simulink library "inp"  (Simulink 7.4)
settings: Solver=ode45  StartTime=0.0  StopTime=10.0  RelTol=1e-3
undefined symbols (not defined in the file): AINP_BrkPedalInterp_X_bar, C_TASK_10MS_S, ENUM_SHIFTER_D, ENUM_SHIFTER_N, ENUM_SHIFTER_P, ENUM_SHIFTER_R, KINP_BonnetCloseVehSpdThre_kph, KINP_EDUCoolantTempFilTm_s, KINP_EDUOilPressureFilTm_s, KINP_EDUOilTempFilTm_s, KINP_EDUSynchDisp_mm, KINP_EDUSynchPosnPWMDC_pct_LowerLimit, KINP_EDUSynchPosnPWMDC_pct_ovrdflg, KINP_EDUSynchPosnPWMDC_pct_ovrdval, KINP_EDUSynchPosnPWMDC_pct_UpperLimit, KINP_ShifterPosConfirmD_s, KINP_ShifterPosConfirmN_s, KINP_ShifterPosConfirmP_s, KINP_ShifterPosConfirmR_s, KINP_SingleAccPedalFltRateLim_pct, KINP_TMSpd2VehSpdSigNeg_rpm, KINP_TMSpd2VehSpdSigPos_rpm, KINP_ValidCheck_EDUSynchPosnPWMDC_dec, KINP_ValidCheck_EDUSynchPosnPWMDC_inc, KINP_ValidCheck_EDUSynchPosnPWMDC_lim, KINP_VehSpdSigKeepThres_kph, KPH2MPS, MIN2SEC, MINP_BrkPedalInterp_pct, MPS2KPH, PI, seat_version_control_block_callbacks, TIRE_RADIUS
libraries: inp_lib x166, hcu_lib x4, simulink x1
(part 9 of 9)

== system inp/INP/INP_10MS/Message (10ms) SCU_HSC_FrP00/Subsystem ==
  VINP_ShifterPosRaw_enum : Inport  OutDataType=fixdt(1, 16)  OutScaling=2^0
  Constant10 : Constant  Value=ENUM_SHIFTER_N  OutDataType=fixdt(1, 16)  OutScaling=2^0
  Constant11 : Constant  Value=ENUM_SHIFTER_R  OutDataType=fixdt(1, 16)  OutScaling=2^0
  Constant22 : Constant  Value=ENUM_SHIFTER_D  OutDataType=fixdt(1, 16)  OutScaling=2^0
  Constant23 : Constant  Value=ENUM_SHIFTER_P  OutDataType=fixdt(1, 16)  OutScaling=2^0
  Constant24 : Constant  Value=KINP_ShifterPosConfirmN_s  OutDataType=fixdt(1, 16)  OutScaling=2^0
  Constant25 : Constant  Value=KINP_ShifterPosConfirmR_s  OutDataType=fixdt(1, 16)  OutScaling=2^0
  Constant26 : Constant  Value=KINP_ShifterPosConfirmD_s  OutDataType=fixdt(1, 16)  OutScaling=2^0
  Constant27 : Constant  Value=KINP_ShifterPosConfirmP_s  OutDataType=fixdt(1, 16)  OutScaling=2^0
  Constant28 : Constant  Value=C_TASK_10MS_S  OutDataTypeMode=single  OutDataType=fixdt(1, 16)  OutScaling=2^0  OutDataTypeStr=single
  Relational Operator{5,10..12} (4 alike) : RelationalOperator  Operator===  LogicOutDataTypeMode=boolean  LogicDataType=fixdt(0, 8)  OutDataTypeStr=boolean
  Relational Operator4 : RelationalOperator  Operator=~=  LogicOutDataTypeMode=boolean  LogicDataType=fixdt(0, 8)  OutDataTypeStr=boolean
  Switch{4,9..12} (5 alike) : Switch  Criteria=u2 ~= 0  Threshold=0.5  OutDataType=fixdt(1, 16)  OutScaling=2^0
  Terminator : Terminator
  Timer : Subsystem
  Unit Delay5 : UnitDelay  X0=ENUM_SHIFTER_P  SampleTime=-1
      settings: AttributesFormatString=Initial value=ENUM_SHIFTER_P
  Unit Delay6 : UnitDelay  SampleTime=-1
  Unit Delay7 : UnitDelay  X0=ENUM_SHIFTER_P  SampleTime=-1
      settings: AttributesFormatString=Initial value=ENUM_SHIFTER_P
  VINP_ShifterPos_enum : Outport  OutDataType=fixdt(1, 16)  OutScaling=2^0
  wires:
  VINP_ShifterPosRaw_enum/1 -> Relational Operator12/1, Relational Operator5/1, Relational Operator11/1, Unit Delay5/1, Relational Operator4/1, Relational Operator10/1, Switch12/1
  Unit Delay5/1 -> Relational Operator4/2
  Constant10/1 -> Relational Operator5/2
  Constant11/1 -> Relational Operator10/2
  Constant22/1 -> Relational Operator11/2
  Constant23/1 -> Relational Operator12/2
  Constant24/1 -> Switch11/1
  Relational Operator5/1 -> Switch11/2
  Constant25/1 -> Switch10/1
  Relational Operator10/1 -> Switch10/2
  Constant26/1 -> Switch4/1
  Relational Operator11/1 -> Switch4/2
  Constant27/1 -> Switch9/1
  Relational Operator12/1 -> Switch9/2
  Switch10/1 -> Switch4/3
  Switch4/1 -> Switch11/3
  Switch11/1 -> Switch9/3
  Switch9/1 -> Unit Delay6/1, Timer/1(To)
  Unit Delay6/1 -> Switch10/3
  Relational Operator4/1 -> Timer/3(reset)
  Constant28/1 -> Timer/2(Ts)
  Timer/1(time) -> Terminator/1
  Timer/2(timeout) -> Switch12/2
  Switch12/1 -> Unit Delay7/1, VINP_ShifterPos_enum/1
  Unit Delay7/1 -> Switch12/3

== system inp/INP/INP_20MS/HW_HCU_20ms/filter ==
  VINP_EDUOilPressureRaw_bar : Inport  OutDataType=sfix(16)  OutScaling=2^0
  Constant : Constant  Value=0.02  OutDataTypeMode=single  OutDataType=fixdt(1, 16)  OutScaling=2^0  OutDataTypeStr=single
  Constant1 : Constant  Value=KINP_EDUOilPressureFilTm_s  OutDataTypeMode=single  OutDataType=fixdt(1, 16)  OutScaling=2^0  OutDataTypeStr=single
  First_Order_Filter : hcu_lib/First_Order_Filter  SystemSampleTime=-1
  VINP_EDUOilPressure_bar : Outport  OutDataType=sfix(16)  OutScaling=2^0
  wires:
  Constant1/1 -> First_Order_Filter/2
  Constant/1 -> First_Order_Filter/3
  First_Order_Filter/1 -> VINP_EDUOilPressure_bar/1
  VINP_EDUOilPressureRaw_bar/1 -> First_Order_Filter/1

== system inp/INP/INP_5MS/HW_HCU_5ms/Subsys VINP_EDUSynchPosnPWMDC_pct ==
  note: Function:
      | 1. Calibration override
      | 2. Valid signal debounce and default value selection
      | 3. High/Low saturation
      | Applicable for:
      | 1. Hardwire analog signals (with corresponding valid flag)
  SigIn : Inport  OutDataType=fixdt(1, 16)  OutScaling=2^0
  SigValidRaw : Inport  Port=2  OutDataType=fixdt(1, 16)  OutScaling=2^0
  srv_ovrdflg : Inport  Port=3  OutDataType=fixdt(1, 16)  OutScaling=2^0
  srv_ovrdval : Inport  Port=4  OutDataType=fixdt(1, 16)  OutScaling=2^0
  Data Type Conversion : DataTypeConversion  OutDataType=fixdt(1, 16)  OutScaling=2^0
  Data Type Conversion1 : DataTypeConversion  OutDataType=fixdt(1, 16)  OutScaling=2^0
  Logical Operator : Logic  Operator=NOT  Inputs=1  AllPortsSameDT=off  OutDataTypeMode=boolean  LogicDataType=fixdt(0, 8)  OutDataTypeStr=boolean
  Logical Operator1 : Logic  Operator=NOT  Inputs=1  AllPortsSameDT=off  OutDataTypeMode=boolean  LogicDataType=fixdt(0, 8)  OutDataTypeStr=boolean
  Logical Operator2 : Logic  Operator=OR  AllPortsSameDT=off  OutDataTypeMode=boolean  OutDataTypeStr=boolean
  MinMax : MinMax  Inputs=2  OutDataType=fixdt(1, 16)  OutScaling=2^0
  MinMax1 : MinMax  Function=max  Inputs=2  OutDataType=fixdt(1, 16)  OutScaling=2^0
  Switch1 : Switch  Criteria=u2 ~= 0  OutDataType=fixdt(1, 16)  OutScaling=2^0
  Switch2 : Switch  Criteria=u2 ~= 0  OutDataType=fixdt(1, 16)  OutScaling=2^0
  Switch3 : Switch  Criteria=u2 ~= 0  Threshold=0.5  OutDataType=sfix(16)  OutScaling=2^0
  Switch4 : Switch  Criteria=u2 ~= 0  Threshold=0.5  OutDataType=sfix(16)  OutScaling=2^0
  Switch5 : Switch  Criteria=u2 ~= 0  Threshold=0.5  OutDataType=sfix(16)  OutScaling=2^0
  Terminator : Terminator
  True : Constant  OutDataTypeMode=boolean  OutDataType=sfix(16)  OutScaling=2^0  OutDataTypeStr=boolean
  Unit Delay : UnitDelay  SampleTime=-1
      settings: AttributesFormatString=Init: %<X0>
  Unit Delay1 : UnitDelay  SampleTime=-1
  rff_ctl : Stateflow chart
  sat : Constant  Value=lim  OutDataTypeMode=uint8  OutDataType=sfix(16)  OutScaling=2^0  OutDataTypeStr=uint8
  sat1 : Constant  Value=inc  OutDataTypeMode=uint8  OutDataType=sfix(16)  OutScaling=2^0  OutDataTypeStr=uint8
  sat2 : Constant  Value=dec  OutDataTypeMode=uint8  OutDataType=sfix(16)  OutScaling=2^0  OutDataTypeStr=uint8
  sat3 : Constant  Value=cal_ovrdflg  OutDataTypeMode=boolean  OutDataType=sfix(16)  OutScaling=2^0  OutDataTypeStr=boolean
  sat4 : Constant  Value=cal_ovrdval  OutDataType=sfix(16)  OutScaling=2^0  OutDataTypeStr=Inherit: Inherit via back propagation
  sat6 : Constant  Value=hi  OutDataType=sfix(16)  OutScaling=2^0  OutDataTypeStr=Inherit: Inherit via back propagation
  sat7 : Constant  Value=lo  OutDataType=sfix(16)  OutScaling=2^0  OutDataTypeStr=Inherit: Inherit via back propagation
  SigOut : Outport  OutDataType=fixdt(1, 16)  OutScaling=2^0
  SigValid : Outport  Port=2  OutDataType=fixdt(1, 16)  OutScaling=2^0
  wires:
  MinMax1/1 -> Switch4/3
  Switch2/1 -> MinMax/1
  sat6/1 -> MinMax/2
  sat7/1 -> MinMax1/2
  MinMax/1 -> MinMax1/1
  [sig_valid] -> Switch5/3
  Logical Operator/1 -> [sig_valid], Switch2/2
  Switch5/1 -> SigValid/1
  True/1 -> Switch5/1
  Logical Operator2/1 -> Switch5/2
  Switch4/1 -> Switch3/3
  Data Type Conversion/1 -> Switch4/1  "cal_ovrdval"
  srv_ovrdval/1 -> Switch3/1  "srv_ovrdval"
  sat3/1 -> Switch4/2, [cal_ovrdflg]  "cal_ovrdflg"
  srv_ovrdflg/1 -> Switch3/2, [service_ovrdflg]  "srv_ovrdflg"
  Switch3/1 -> SigOut/1, Unit Delay1/1
  [service_ovrdflg] -> Logical Operator2/1
  [cal_ovrdflg] -> Logical Operator2/2
  SigValidRaw/1 -> Logical Operator1/1, Switch1/2
  Logical Operator1/1 -> rff_ctl/4(i_fault)
  Unit Delay/1 -> Switch1/3
  Switch1/1 -> Switch2/1, Unit Delay/1
  Data Type Conversion1/1 -> Switch2/3
  rff_ctl/2(ff_count) -> Terminator/1
  rff_ctl/1(fault_flg) -> Logical Operator/1
  sat2/1 -> rff_ctl/3(dec)
  sat1/1 -> rff_ctl/2(inc)
  sat/1 -> rff_ctl/1(sat)
  SigIn/1 -> Switch1/1
  sat4/1 -> Data Type Conversion/1
  Unit Delay1/1 -> Data Type Conversion1/1

== system inp/INP/Pre-Process/BINP_ouputs_100ms/Outputs_100ms ==
  VINP_BonnetOpen_flg : Inport  OutDataType=fixdt(1, 16)  OutScaling=2^0
  BINP_rawoutputs_100ms : Inport  Port=2  OutDataType=fixdt(1, 16)  OutScaling=2^0
  Bus Creator1 : BusCreator  Inputs=5
  Bus Creator2 : BusCreator  Inputs=9
  Bus Selector1 : BusSelector  OutputSignals=BINP_ISC_HSC2_FrP05,BINP_TC_HSC2_FrP03,BINP_ISC_HSC2_FrP01,BINP_ISC_HSC2_FrP02,BINP_PMU_HSC_FrP00,BINP_SMU_HSC_FrP07,BINP_SMU_HSC_FrP00,BINP_HW_HCU_100ms
  Bus Selector2 : BusSelector  OutputSignals=BINP_SMU_HSC_FrP06.VINP_DriverDoorOpen_flg,BINP_SMU_HSC_FrP06.VINP_ATCEngOnReq_enum,BINP_SMU_HSC_FrP06.VINP_ACCompressorPower_kW,BINP_SMU_HSC_FrP06.VINP_SMUHSCFrP06Active_flg
  Bus Selector7 : BusSelector  OutputSignals=BINP_ISC_HSC2_FrP05,BINP_TC_HSC2_FrP03,BINP_ISC_HSC2_FrP01,BINP_ISC_HSC2_FrP02,BINP_PMU_HSC_FrP00,BINP_SMU_HSC_FrP07,BINP_SMU_HSC_FrP00,BINP_HW_HCU_100ms,BINP_SMU_HSC_FrP06  OutputAsBus=on
  BINP_outputs_100ms : Outport  OutDataType=fixdt(1, 16)  OutScaling=2^0
  wires:
  Bus Creator1/1 -> Bus Creator2/9  "BINP_SMU_HSC_FrP06"
  Bus Selector1/8 -> Bus Creator2/8  "<BINP_HW_HCU_100ms>"
  Bus Selector1/7 -> Bus Creator2/7  "<BINP_SMU_HSC_FrP00>"
  Bus Selector1/6 -> Bus Creator2/6  "<BINP_SMU_HSC_FrP07>"
  Bus Selector1/5 -> Bus Creator2/5  "<BINP_PMU_HSC_FrP00>"
  Bus Selector1/4 -> Bus Creator2/4  "<BINP_ISC_HSC2_FrP02>"
  Bus Selector1/3 -> Bus Creator2/3  "<BINP_ISC_HSC2_FrP01>"
  Bus Selector1/2 -> Bus Creator2/2  "<BINP_TC_HSC2_FrP03>"
  Bus Selector1/1 -> Bus Creator2/1  "<BINP_ISC_HSC2_FrP05>"
  VINP_BonnetOpen_flg/1 -> Bus Creator1/5
  Bus Selector2/4 -> Bus Creator1/4  "<VINP_SMUHSCFrP06Active_flg>"
  Bus Selector2/3 -> Bus Creator1/3  "<VINP_ACCompressorPower_kW>"
  Bus Selector2/2 -> Bus Creator1/2  "<VINP_ATCEngOnReq_enum>"
  Bus Selector2/1 -> Bus Creator1/1  "<VINP_DriverDoorOpen_flg>"
  Bus Creator2/1 -> Bus Selector7/1
  Bus Selector7/1 -> BINP_outputs_100ms/1  "BINP_outputs_100ms"
  BINP_rawoutputs_100ms/1 -> Bus Selector2/1, Bus Selector1/1

== system inp/INP/Pre-Process/BINP_ouputs_100ms/Signal Process ==
  VINP_VehSpd_kph : Inport  OutDataType=fixdt(1, 16)  OutScaling=2^0
  VINP_BonnetOpenRaw_flg : Inport  Port=2  OutDataType=fixdt(1, 16)  OutScaling=2^0
  VINP_BonnetOpenRawValid_flg : Inport  Port=3  OutDataType=fixdt(1, 16)  OutScaling=2^0
  trig_sig_chk : TriggerPort  TriggerType=function-call
  Abs : Abs  OutDataType=fixdt(1, 16)  OutScaling=2^0
  Constant : Constant  Value=KINP_BonnetCloseVehSpdThre_kph  OutDataType=fixdt(1, 16)  OutScaling=2^0
  Relational Operator : RelationalOperator  Operator=<=  LogicOutDataTypeMode=boolean  LogicDataType=fixdt(0, 8)  OutDataTypeStr=boolean
  Switch : Switch  Criteria=u2 ~= 0  Threshold=0.5  OutDataType=fixdt(1, 16)  OutScaling=2^0
  VINP_BonnetOpen_flg : Outport  OutDataType=fixdt(1, 16)  OutScaling=2^0
  wires:
  Abs/1 -> Relational Operator/1
  Switch/1 -> VINP_BonnetOpen_flg/1  "VINP_BonnetOpen_flg"
  Relational Operator/1 -> Switch/3
  Constant/1 -> Relational Operator/2
  VINP_VehSpd_kph/1 -> Abs/1
  VINP_BonnetOpenRaw_flg/1 -> Switch/1
  VINP_BonnetOpenRawValid_flg/1 -> Switch/2

== system inp/INP/Pre-Process/BINP_ouputs_10ms/Signal Process ==
  BINP_rawoutputs_10ms : Inport  OutDataType=sfix(16)  OutScaling=2^0
  VDSM_SngAccPedInvldFlt_flg : Inport  Port=2  OutDataType=sfix(16)  OutScaling=2^0
  trig_sig_chk : TriggerPort  TriggerType=function-call
  Bus Selector1 : BusSelector  OutputSignals=BINP_EMS_HSC_FrP00.VINP_EngSpdRaw_rpm,BINP_EMS_HSC_FrP00.VINP_EngSpdRawValid_flg,BINP_ISC_HSC2_FrP03.VINP_ISGSpdRaw_rpm,BINP_ISC_HSC2_FrP03.VINP_ISGSpdRawValid_flg
  Bus Selector2 : BusSelector  OutputSignals=BINP_ISC_HSC2_FrP03.VINP_ISGSpdRaw_rpm,BINP_ISC_HSC2_FrP03.VINP_ISGSpdRawValid_flg,BINP_EMS_HSC_FrP00.VINP_EngSpdRaw_rpm,BINP_EMS_HSC_FrP00.VINP_EngSpdRawValid_flg
  Bus Selector3 : BusSelector  OutputSignals=BINP_ISC_HSC2_FrP03.VINP_ISGSpdRawValid_flg,BINP_EMS_HSC_FrP00.VINP_EngSpdRawValid_flg
  Bus Selector4 : BusSelector  OutputSignals=BINP_ISC_HSC2_FrP03.VINP_ISGSpdRawValid_flg,BINP_EMS_HSC_FrP00.VINP_EngSpdRawValid_flg
  Bus Selector5 : BusSelector  OutputSignals=BINP_EMS_HSC_FrP07.VINP_AccelPedalPosnRaw_pct
  Constant : Constant  Value=0  OutDataTypeMode=single  OutDataType=fixdt(1, 16)  OutScaling=2^0  OutDataTypeStr=single
  Constant1 : Constant  Value=0  OutDataTypeMode=single  OutDataType=fixdt(1, 16)  OutScaling=2^0  OutDataTypeStr=single
  IncFilter : Subsystem
  Logical Operator : Logic  Operator=OR  AllPortsSameDT=off  OutDataTypeMode=boolean  LogicDataType=fixdt(0, 8)  OutDataTypeStr=boolean
  Logical Operator1 : Logic  Operator=OR  AllPortsSameDT=off  OutDataTypeMode=boolean  LogicDataType=fixdt(0, 8)  OutDataTypeStr=boolean
  Switch{,1..3} (4 alike) : Switch  Criteria=u2 ~= 0  Threshold=0.5  OutDataType=fixdt(1, 16)  OutScaling=2^0
  cnst_ValidCheck_EngCoolantTemp : Constant  Value=KINP_SingleAccPedalFltRateLim_pct  OutDataTypeMode=single  OutDataType=sfix(16)  OutScaling=2^0  OutDataTypeStr=single
  VINP_EngSpd_rpm : Outport  OutDataType=sfix(16)  OutScaling=2^0
  VINP_EngSpdValid_flg : Outport  Port=2  OutDataType=sfix(16)  OutScaling=2^0
  VINP_ISGSpd_rpm : Outport  Port=3  OutDataType=sfix(16)  OutScaling=2^0
  VINP_ISGSpdValid_flg : Outport  Port=4  OutDataType=sfix(16)  OutScaling=2^0
  VINP_AccelPedalPosn_pct : Outport  Port=5  OutDataType=sfix(16)  OutScaling=2^0
  wires:
  Bus Selector3/2 -> Logical Operator/2  "<VINP_EngSpdRawValid_flg>"
  Bus Selector3/1 -> Logical Operator/1  "<VINP_ISGSpdRawValid_flg>"
  Switch2/1 -> VINP_ISGSpd_rpm/1  "VINP_ISGSpd_rpm"
  Switch/1 -> VINP_EngSpd_rpm/1  "VINP_EngSpd_rpm"
  Switch3/1 -> Switch2/3
  Bus Selector2/4 -> Switch3/2  "<VINP_EngSpdRawValid_flg>"
  Bus Selector2/3 -> Switch3/1  "<VINP_EngSpdRaw_rpm>"
  Bus Selector2/2 -> Switch2/2  "<VINP_ISGSpdRawValid_flg>"
  Bus Selector2/1 -> Switch2/1  "<VINP_ISGSpdRaw_rpm>"
  Constant1/1 -> Switch3/3
  Constant/1 -> Switch1/3
  Switch1/1 -> Switch/3
  Bus Selector1/3 -> Switch1/1  "<VINP_ISGSpdRaw_rpm>"
  Bus Selector1/4 -> Switch1/2  "<VINP_ISGSpdRawValid_flg>"
  Bus Selector1/1 -> Switch/1  "<VINP_EngSpdRaw_rpm>"
  Bus Selector1/2 -> Switch/2  "<VINP_EngSpdRawValid_flg>"
  BINP_rawoutputs_10ms/1 -> Bus Selector2/1, Bus Selector3/1, Bus Selector4/1, Bus Selector5/1, Bus Selector1/1
  Logical Operator/1 -> VINP_EngSpdValid_flg/1  "VINP_EngSpdValid_flg"
  Bus Selector4/1 -> Logical Operator1/1  "<VINP_ISGSpdRawValid_flg>"
  Bus Selector4/2 -> Logical Operator1/2  "<VINP_EngSpdRawValid_flg>"
  Logical Operator1/1 -> VINP_ISGSpdValid_flg/1  "VINP_ISGSpdValid_flg"
  VDSM_SngAccPedInvldFlt_flg/1 -> IncFilter/4(Fault)
  Bus Selector5/1 -> IncFilter/1(Raw), IncFilter/2(Init)  "<VINP_AccelPedalPosnRaw_pct>"
  IncFilter/1(Fil) -> VINP_AccelPedalPosn_pct/1  "VINP_AccelPedalPosn_pct"
  cnst_ValidCheck_EngCoolantTemp/1 -> IncFilter/3(RateLimit)

== system inp/INP/Pre-Process/BINP_ouputs_10ms/outputs_10ms ==
  BINP_rawoutputs_10ms : Inport
  VINP_VehSpd_kph : Inport  Port=2
  VINP_VehSpdValid_flg : Inport  Port=3
  VINP_EngSpd_rpm : Inport  Port=4
  VINP_EngSpdValid_flg : Inport  Port=5
  VINP_ISGSpd_rpm : Inport  Port=6
  VINP_ISGSpdValid_flg : Inport  Port=7
  VINP_AccelPedalPosn_pct : Inport  Port=8
  Bus Creator1 : BusCreator  Inputs=6
  Bus Creator2 : BusCreator  Inputs=12
  Bus Creator3 : BusCreator  Inputs=14
  Bus Creator4 : BusCreator  Inputs=14
  Bus Creator5 : BusCreator  Inputs=8
  Bus Selector1 : BusSelector  OutputSignals=BINP_ABS_DSC_HSC_FrP00.VINP_WheelRoughRoad_mps2,BINP_ABS_DSC_HSC_FrP00.VINP_WheelRoughRoadValid_flg,BINP_ABS_DSC_HSC_FrP00.VINP_ABSDSCHSCFrP00Active_flg,BINP_ABS_DSC_HSC_FrP00.VINP_VehSpdRawValid_flg
  Bus Selector2 : BusSelector  OutputSignals=BINP_DSC_HSC_FrP00,BINP_DSC_HSC_FrP02,BINP_SCU_HSC_FrP00,BINP_ABS_DSC_HSC_FrP03,BINP_TC_HSC2_FrP01,BINP_ISC_HSC2_FrP04,BINP_HW_HCU_10ms
  Bus Selector3 : BusSelector  OutputSignals=BINP_EMS_HSC_FrP00.VINP_BrkLightSwitchActive_flg,BINP_EMS_HSC_FrP00.VINP_BrkLightSwitchActiveValid_flg,BINP_EMS_HSC_FrP00.VINP_EngTqFriction_Nm,BINP_EMS_HSC_FrP00.VINP_EngTqIndAct_Nm,BINP_EMS_HSC_FrP00.VINP_EngTqIndActValid_flg,BINP_EMS_HSC_FrP00.VINP_EngTqStandard_Nm,BINP_EMS_HSC_FrP00.VINP_CruiseTqReq_Nm,BINP_EMS_HSC_FrP00.VINP_EngTqModelStatus_enum,BINP_EMS_HSC_FrP00.VINP_KeySwitchStateIGN_flg,BINP_EMS_HSC_FrP00.VINP_EMSHSCFrP00Active_flg,BINP_EMS_HSC_FrP00.VINP_BrkLightSWPUnlockActive_flg,BINP_EMS_HSC_FrP00.VINP_BrkLightSWPUnlockActiveValid_flg
  Bus Selector4 : BusSelector  OutputSignals=BINP_ISC_HSC2_FrP03.VINP_ISGACShortCircReady_flg,BINP_ISC_HSC2_FrP03.VINP_ISGDiagReq_flg,BINP_ISC_HSC2_FrP03.VINP_ISGMode_enum,BINP_ISC_HSC2_FrP03.VINP_ISGTqAct_Nm,BINP_ISC_HSC2_FrP03.VINP_ISGTqActValid_flg,BINP_ISC_HSC2_FrP03.VINP_ISCHSC2FrP03Active_flg
  Bus Selector5 : BusSelector  OutputSignals=BINP_TC_HSC2_FrP02
  Bus Selector6 : BusSelector  OutputSignals=BINP_EMS_HSC_FrP07.VINP_EngSpdMon_rpm,BINP_EMS_HSC_FrP07.VINP_EngStartComplete_flg,BINP_EMS_HSC_FrP07.VINP_EngStopped_flg,BINP_EMS_HSC_FrP07.VINP_EngTqAllowedMinMon_Nm,BINP_EMS_HSC_FrP07.VINP_EngTqMax_Nm,BINP_EMS_HSC_FrP07.VINP_EngTqMin_Nm,BINP_EMS_HSC_FrP07.VINP_FuelCutActive_flg,BINP_EMS_HSC_FrP07.VINP_LamdLoopActive_flg,BINP_EMS_HSC_FrP07.VINP_EngIdle_flg,BINP_EMS_HSC_FrP07.VINP_AccelPedalPosnValid_flg,BINP_EMS_HSC_FrP07.VINP_EMSFltLevel_enum,BINP_EMS_HSC_FrP07.VINP_CatLightOffReq_flg,BINP_EMS_HSC_FrP07.VINP_EMSHSCFrP07Active_flg
  Bus Selector7 : BusSelector  OutputSignals=BINP_TC_HSC2_FrP02,BINP_EMS_HSC_FrP00,BINP_EMS_HSC_FrP07,BINP_ABS_DSC_HSC_FrP00,BINP_DSC_HSC_FrP00,BINP_DSC_HSC_FrP02,BINP_SCU_HSC_FrP00,BINP_ABS_DSC_HSC_FrP03,BINP_TC_HSC2_FrP01,BINP_ISC_HSC2_FrP03,BINP_ISC_HSC2_FrP04,BINP_HW_HCU_10ms  OutputAsBus=on
  BINP_outputs_10ms : Outport
  wires:
  Bus Creator1/1 -> Bus Creator2/10  "BINP_ABS_DSC_HSC_FrP00"
  Bus Selector2/7 -> Bus Creator2/9  "<BINP_HW_HCU_10ms>"
  Bus Selector2/6 -> Bus Creator2/8  "<BINP_ISC_HSC2_FrP04>"
  Bus Selector2/5 -> Bus Creator2/7  "<BINP_TC_HSC2_FrP01>"
  Bus Selector2/4 -> Bus Creator2/6  "<BINP_ABS_DSC_HSC_FrP03>"
  Bus Selector2/3 -> Bus Creator2/5  "<BINP_SCU_HSC_FrP00>"
  Bus Selector2/2 -> Bus Creator2/4  "<BINP_DSC_HSC_FrP02>"
  Bus Selector2/1 -> Bus Creator2/3  "<BINP_DSC_HSC_FrP00>"
  Bus Creator5/1 -> Bus Creator2/12  "BINP_ISC_HSC2_FrP03"
  Bus Creator3/1 -> Bus Creator2/11  "BINP_EMS_HSC_FrP00"
  VINP_ISGSpdValid_flg/1 -> Bus Creator5/8  "VINP_ISGSpdValid_flg"
  VINP_ISGSpd_rpm/1 -> Bus Creator5/7  "VINP_ISGSpd_rpm"
  Bus Selector4/6 -> Bus Creator5/6  "<VINP_ISCHSC2FrP03Active_flg>"
  Bus Selector4/5 -> Bus Creator5/5  "<VINP_ISGTqActValid_flg>"
  Bus Selector4/4 -> Bus Creator5/4  "<VINP_ISGTqAct_Nm>"
  Bus Selector4/3 -> Bus Creator5/3  "<VINP_ISGMode_enum>"
  Bus Selector4/2 -> Bus Creator5/2  "<VINP_ISGDiagReq_flg>"
  Bus Selector4/1 -> Bus Creator5/1  "<VINP_ISGACShortCircReady_flg>"
  VINP_EngSpdValid_flg/1 -> Bus Creator3/14  "VINP_EngSpdValid_flg"
  VINP_EngSpd_rpm/1 -> Bus Creator3/13  "VINP_EngSpd_rpm"
  Bus Selector3/12 -> Bus Creator3/12  "<VINP_BrkLightSWPUnlockActiveValid_flg>"
  Bus Selector3/11 -> Bus Creator3/11  "<VINP_BrkLightSWPUnlockActive_flg>"
  Bus Selector3/10 -> Bus Creator3/10  "<VINP_EMSHSCFrP00Active_flg>"
  Bus Selector3/9 -> Bus Creator3/9  "<VINP_KeySwitchStateIGN_flg>"
  Bus Selector3/8 -> Bus Creator3/8  "<VINP_EngTqModelStatus_enum>"
  Bus Selector3/7 -> Bus Creator3/7  "<VINP_CruiseTqReq_Nm>"
  Bus Selector3/6 -> Bus Creator3/6  "<VINP_EngTqStandard_Nm>"
  Bus Selector3/5 -> Bus Creator3/5  "<VINP_EngTqIndActValid_flg>"
  Bus Selector3/4 -> Bus Creator3/4  "<VINP_EngTqIndAct_Nm>"
  Bus Selector3/3 -> Bus Creator3/3  "<VINP_EngTqFriction_Nm>"
  Bus Selector3/2 -> Bus Creator3/2  "<VINP_BrkLightSwitchActiveValid_flg>"
  Bus Selector3/1 -> Bus Creator3/1  "<VINP_BrkLightSwitchActive_flg>"
  Bus Selector7/1 -> BINP_outputs_10ms/1  "BINP_outputs_10ms"
  Bus Selector1/3 -> Bus Creator1/3  "<VINP_ABSDSCHSCFrP00Active_flg>"
  Bus Selector1/2 -> Bus Creator1/2  "<VINP_WheelRoughRoadValid_flg>"
  Bus Selector1/1 -> Bus Creator1/1  "<VINP_WheelRoughRoad_mps2>"
  BINP_rawoutputs_10ms/1 -> Bus Selector1/1, Bus Selector4/1, Bus Selector3/1, Bus Selector2/1, Bus Selector5/1, Bus Selector6/1
  Bus Creator2/1 -> Bus Selector7/1
  Bus Selector1/4 -> Bus Creator1/4  "<VINP_VehSpdRawValid_flg>"
  VINP_VehSpd_kph/1 -> Bus Creator1/5
  VINP_VehSpdValid_flg/1 -> Bus Creator1/6
  Bus Selector5/1 -> Bus Creator2/1  "<BINP_TC_HSC2_FrP02>"
  Bus Creator4/1 -> Bus Creator2/2  "BINP_EMS_HSC_FrP07"
  Bus Selector6/1 -> Bus Creator4/1  "<VINP_EngSpdMon_rpm>"
  Bus Selector6/2 -> Bus Creator4/2  "<VINP_EngStartComplete_flg>"
  Bus Selector6/3 -> Bus Creator4/3  "<VINP_EngStopped_flg>"
  Bus Selector6/4 -> Bus Creator4/4  "<VINP_EngTqAllowedMinMon_Nm>"
  Bus Selector6/5 -> Bus Creator4/5  "<VINP_EngTqMax_Nm>"
  Bus Selector6/6 -> Bus Creator4/6  "<VINP_EngTqMin_Nm>"
  Bus Selector6/7 -> Bus Creator4/7  "<VINP_FuelCutActive_flg>"
  Bus Selector6/8 -> Bus Creator4/8  "<VINP_LamdLoopActive_flg>"
  Bus Selector6/9 -> Bus Creator4/9  "<VINP_EngIdle_flg>"
  Bus Selector6/10 -> Bus Creator4/10  "<VINP_AccelPedalPosnValid_flg>"
  Bus Selector6/11 -> Bus Creator4/12  "<VINP_EMSFltLevel_enum>"
  Bus Selector6/12 -> Bus Creator4/13  "<VINP_CatLightOffReq_flg>"
  Bus Selector6/13 -> Bus Creator4/14  "<VINP_EMSHSCFrP07Active_flg>"
  VINP_AccelPedalPosn_pct/1 -> Bus Creator4/11

== system inp/INP/Pre-Process/BINP_ouputs_5ms/Outputs_5ms ==
  BINP_rawoutputs_5ms : Inport  OutDataType=fixdt(1, 16)  OutScaling=2^0
  VINP_EDUOutputShaftSpd_rpm : Inport  Port=2  OutDataType=fixdt(1, 16)  OutScaling=2^0
  VINP_EDUOutputShaftSpdRawValid_flg : Inport  Port=3  OutDataType=fixdt(1, 16)  OutScaling=2^0
  VINP_EDUSynchPosn_mm : Inport  Port=4  OutDataType=fixdt(1, 16)  OutScaling=2^0
  VINP_EDUSynchPosnValid_flg : Inport  Port=5  OutDataType=fixdt(1, 16)  OutScaling=2^0
  Bus Creator2 : BusCreator  Inputs=9
  Bus Selector1 : BusSelector  OutputSignals=BINP_HardwireInputs.VINP_EDUSynchPosnPWMKDC_pct,BINP_HardwireInputs.VINP_EDUSynchPosnPWMKDCValid_flg,BINP_HardwireInputs.VINP_EDUSynchPosnPWMDC_pct,BINP_HardwireInputs.VINP_EDUSynchPosnPWMDCValid_flg,BINP_HardwireInputs.VINP_EDUOutputShaftSpdRawValid_flg
  Bus Selector7 : BusSelector  OutputSignals=VINP_EDUOutputShaftSpd_rpm,VINP_EDUOutputShaftSpdValid_flg,VINP_EDUSynchPosnPWMKDC_pct,VINP_EDUSynchPosnPWMKDCValid_flg,VINP_EDUSynchPosn_mm,VINP_EDUSynchPosnValid_flg,VINP_EDUSynchPosnPWMDC_pct,VINP_EDUSynchPosnPWMDCValid_flg,VINP_EDUOutputShaftSpdRawValid_flg  OutputAsBus=on
  BINP_outputs_5ms : Outport  OutDataType=fixdt(1, 16)  OutScaling=2^0
  wires:
  Bus Creator2/1 -> Bus Selector7/1
  Bus Selector1/4 -> Bus Creator2/4  "<VINP_EDUSynchPosnPWMDCValid_flg>"
  Bus Selector1/3 -> Bus Creator2/3  "<VINP_EDUSynchPosnPWMDC_pct>"
  Bus Selector1/2 -> Bus Creator2/2  "<VINP_EDUSynchPosnPWMKDCValid_flg>"
  Bus Selector1/1 -> Bus Creator2/1  "<VINP_EDUSynchPosnPWMKDC_pct>"
  Bus Selector7/1 -> BINP_outputs_5ms/1  "BINP_outputs_5ms"
  BINP_rawoutputs_5ms/1 -> Bus Selector1/1
  Bus Selector1/5 -> Bus Creator2/5  "<VINP_EDUOutputShaftSpdRawValid_flg>"
  VINP_EDUOutputShaftSpd_rpm/1 -> Bus Creator2/6
  VINP_EDUOutputShaftSpdRawValid_flg/1 -> Bus Creator2/7
  VINP_EDUSynchPosn_mm/1 -> Bus Creator2/8
  VINP_EDUSynchPosnValid_flg/1 -> Bus Creator2/9

== system inp/INP/Pre-Process/BINP_ouputs_5ms/Signal Process ==
  VINP_EDUSynchPosnPWMKDC_pct : Inport  OutDataType=sfix(16)  OutScaling=2^0
  VINP_EDUSynchPosnPWMKDCValid_flg : Inport  Port=2  OutDataType=sfix(16)  OutScaling=2^0
  VINP_EDUSynchPosnPWMDC_pct : Inport  Port=3  OutDataType=sfix(16)  OutScaling=2^0
  VINP_EDUSynchPosnPWMDCValid_flg : Inport  Port=4  OutDataType=sfix(16)  OutScaling=2^0
  VINP_EDUOutputShaftSpdRaw_rpm : Inport  Port=5  OutDataType=sfix(16)  OutScaling=2^0
  VINP_EDUOutputShaftSpdRawValid_flg : Inport  Port=6  OutDataType=sfix(16)  OutScaling=2^0
  VINP_VehSpdRawABS_kph : Inport  Port=7  OutDataType=sfix(16)  OutScaling=2^0
  VINP_VehSpdRawValid_flg : Inport  Port=8  OutDataType=sfix(16)  OutScaling=2^0
  VINP_TMSpd_rpm : Inport  Port=9  OutDataType=sfix(16)  OutScaling=2^0
  trig_sig_chk : TriggerPort  TriggerType=function-call
  SynchPosn : Subsystem
      settings: RTWSystemCode=Inline
  VehSpdRaw_Calc : Subsystem
  VehSpd_Calc : Subsystem
      settings: RTWSystemCode=Inline
  VINP_EDUOutputShaftSpd_rpm : Outport  OutDataType=sfix(16)  OutScaling=2^0
  VINP_EDUOutputShaftSpdValid_flg : Outport  Port=2  OutDataType=sfix(16)  OutScaling=2^0
  VINP_EDUSynchPosn_mm : Outport  Port=3  OutDataType=sfix(16)  OutScaling=2^0
  VINP_EDUSynchPosnValid_flg : Outport  Port=4  OutDataType=sfix(16)  OutScaling=2^0
  VINP_VehSpd_kph : Outport  Port=5  OutDataType=sfix(16)  OutScaling=2^0
  VINP_VehSpdValid_flg : Outport  Port=6  OutDataType=sfix(16)  OutScaling=2^0
  wires:
  VehSpdRaw_Calc/1(VINP_VehSpdRaw_kph) -> VehSpd_Calc/2(<VINP_VehSpdRaw_kph>)
  VINP_VehSpdRawABS_kph/1 -> VehSpdRaw_Calc/2(VINP_VehSpdRawABS_kph)
  VINP_EDUOutputShaftSpdRawValid_flg/1 -> VehSpd_Calc/3(VINP_EDUOutputShaftSpdRawValid_flg), VehSpdRaw_Calc/4(VINP_EDUOutputShaftSpdRawValid_flg)
  VINP_EDUOutputShaftSpdRaw_rpm/1 -> VehSpd_Calc/1(VINP_EDUOutputShaftSpdRaw_rpm), VehSpdRaw_Calc/1(VINP_EDUOutputShaftSpdRaw_rpm)
  VINP_TMSpd_rpm/1 -> VehSpdRaw_Calc/3(VINP_TMSpd_rpm)
  VehSpd_Calc/4(VINP_EDUOutputShaftSpdValid_flg) -> VINP_EDUOutputShaftSpdValid_flg/1
  VehSpd_Calc/3(VINP_VehSpdValid_flg) -> VINP_VehSpdValid_flg/1
  VehSpd_Calc/2(VINP_EDUOutputShaftSpd_rpm) -> VINP_EDUOutputShaftSpd_rpm/1
  VehSpd_Calc/1(VINP_VehSpd_kph) -> VINP_VehSpd_kph/1
  SynchPosn/2(VINP_EDUSynchPosnValid_flg) -> VINP_EDUSynchPosnValid_flg/1
  SynchPosn/1(VINP_EDUSynchPosn_mm) -> VINP_EDUSynchPosn_mm/1
  VINP_VehSpdRawValid_flg/1 -> VehSpd_Calc/4(<VINP_VehSpdRawValid_flg>)
  VINP_EDUSynchPosnPWMDCValid_flg/1 -> SynchPosn/4(VINP_EDUSynchPosnPWMDCValid_flg)
  VINP_EDUSynchPosnPWMDC_pct/1 -> SynchPosn/3(VINP_EDUSynchPosnPWMDC_pct)
  VINP_EDUSynchPosnPWMKDCValid_flg/1 -> SynchPosn/2(VINP_EDUSynchPosnPWMKDCValid_flg)
  VINP_EDUSynchPosnPWMKDC_pct/1 -> SynchPosn/1(VINP_EDUSynchPosnPWMKDC_pct)

== system inp/INP/INP_10MS/Message (10ms) SCU_HSC_FrP00/Subsystem/Timer ==
  note: /* avoid eps error */
  To : Inport
  Ts : Inport  Port=2
  reset : Inport  Port=3
  Add1 : Sum  OutDataType=fixdt(1, 16)  OutScaling=2^-10
  Add2 : Sum  OutDataType=fixdt(1, 16)  OutScaling=2^-10
  Constant : Constant  Value=0  OutDataTypeMode=single  OutDataType=sfix(16)  OutScaling=2^0  OutDataTypeStr=single
  Constant1 : Constant  Value=0  OutDataTypeMode=boolean  OutDataType=sfix(16)  OutScaling=2^0  OutDataTypeStr=boolean
  Gain3 : Gain  Gain=0.5  ParameterDataType=fixdt(1, 16)  ParameterScaling=2^0  OutDataType=fixdt(1, 16)  OutScaling=2^0
  Relational Operator1 : RelationalOperator  Operator=>  LogicOutDataTypeMode=boolean  LogicDataType=fixdt(0, 8)  OutDataTypeStr=boolean
  Switch1 : Switch  Criteria=u2 ~= 0  Threshold=0.5  OutDataType=fixdt(1, 16)  OutScaling=2^0
      settings: AttributesFormatString=<criteria=%<criteria>>\n<threshold=%<threshold>>
  Switch2 : Switch  Criteria=u2 ~= 0  Threshold=0.5  OutDataType=fixdt(1, 16)  OutScaling=2^0
      settings: AttributesFormatString=<criteria=%<criteria>>\n<threshold=%<threshold>>
  Unit Delay1 : UnitDelay  SampleTime=-1
      settings: AttributesFormatString=<initial=%<x0>>\n<tsample=%<sampleTime>>
  time : Outport
  timeout : Outport  Port=2
  wires:
  Constant1/1 -> Switch1/1
  [Reset] -> Switch1/2
  Switch1/1 -> timeout/1
  Relational Operator1/1 -> Switch1/3
  reset/1 -> [Reset], Switch2/2
  Unit Delay1/1 -> Add2/2
  Ts/1 -> [Ts]
  [Ts] -> Gain3/1
  [Ts] -> Add2/1
  Add2/1 -> Switch2/3
  Constant/1 -> Switch2/1
  Switch2/1 -> [Tv], time/1, Unit Delay1/1
  Gain3/1 -> Add1/2
  [Tv] -> Add1/1
  Add1/1 -> Relational Operator1/1
  To/1 -> Relational Operator1/2

== system inp/INP/Pre-Process/BINP_ouputs_10ms/Signal Process/IncFilter ==
  Raw : Inport  OutDataType=sfix(16)  OutScaling=2^0
  Init : Inport  Port=2  OutDataType=sfix(16)  OutScaling=2^0
  RateLimit : Inport  Port=3  OutDataType=sfix(16)  OutScaling=2^0
  Fault : Inport  Port=4  OutDataType=sfix(16)  OutScaling=2^0
  Const4 : Constant  Value=0  OutDataTypeMode=boolean  OutDataType=sfix(16)  OutScaling=2^0  OutDataTypeStr=boolean
  Logical Operator1 : Logic  AllPortsSameDT=off  OutDataTypeMode=boolean  LogicDataType=fixdt(0, 8)  OutDataTypeStr=boolean
  Relational Operator : RelationalOperator  LogicOutDataTypeMode=boolean  OutDataTypeStr=boolean
  Sum1 : Sum  OutDataType=sfix(16)  OutScaling=2^0
  Sum4 : Sum  Inputs=+-  OutDataType=sfix(16)  OutScaling=2^0
  Switch1 : Switch  Criteria=u2 ~= 0  OutDataType=sfix(16)  OutScaling=2^0
  Switch3 : Switch  Criteria=u2 ~= 0  OutDataType=sfix(16)  OutScaling=2^0
  delay : UnitDelay  SampleTime=-1
  delay1 : UnitDelay  X0=1  SampleTime=-1
  Fil : Outport  OutDataType=sfix(16)  OutScaling=2^0
  wires:
  Sum1/1 -> Switch3/1
  Sum4/1 -> Relational Operator/1
  RateLimit/1 -> Sum1/1, Relational Operator/2
  Switch3/1 -> Fil/1, delay/1
  Raw/1 -> Sum4/1, Switch3/3
  Switch1/1 -> Sum1/2, Sum4/2
  Const4/1 -> delay1/1
  delay1/1 -> Switch1/2
  Init/1 -> Switch1/1
  delay/1 -> Switch1/3
  Relational Operator/1 -> Logical Operator1/1
  Logical Operator1/1 -> Switch3/2
  Fault/1 -> Logical Operator1/2

== system inp/INP/Pre-Process/BINP_ouputs_5ms/Signal Process/SynchPosn ==
  VINP_EDUSynchPosnPWMKDC_pct : Inport  OutDataType=sfix(16)  OutScaling=2^0
  VINP_EDUSynchPosnPWMKDCValid_flg : Inport  Port=2  OutDataType=sfix(16)  OutScaling=2^0
  VINP_EDUSynchPosnPWMDC_pct : Inport  Port=3  OutDataType=sfix(16)  OutScaling=2^0
  VINP_EDUSynchPosnPWMDCValid_flg : Inport  Port=4  OutDataType=sfix(16)  OutScaling=2^0
  Constant2 : Constant  Value=KINP_EDUSynchDisp_mm  OutDataType=fixdt(1, 16)  OutScaling=2^0
  Gain : Gain  Gain=-1  ParameterDataType=fixdt(1, 16)  ParameterScaling=2^0  OutDataType=fixdt(1, 16)  OutScaling=2^0
  Logical Operator : Logic  AllPortsSameDT=off  OutDataTypeMode=boolean  OutDataTypeStr=boolean
  Logical Operator1 : Logic  Operator=NOT  AllPortsSameDT=off  OutDataTypeMode=boolean  OutDataTypeStr=boolean
  Logical Operator2 : Logic  AllPortsSameDT=off  OutDataTypeMode=boolean  OutDataTypeStr=boolean
  Logical Operator3 : Logic  Operator=NOT  AllPortsSameDT=off  OutDataTypeMode=boolean  OutDataTypeStr=boolean
  Switch1 : Switch  Criteria=u2 ~= 0  Threshold=0.5  OutDataType=sfix(16)  OutScaling=2^0
  Switch2 : Switch  Criteria=u2 ~= 0  Threshold=0.5  OutDataType=sfix(16)  OutScaling=2^0
  cnst_EDUSynchDisp : Constant  Value=KINP_EDUSynchDisp_mm  OutDataType=fixdt(1, 16)  OutScaling=2^0
  pct2mm1 : Subsystem  TreatAsAtomicUnit=on
      settings: RTWSystemCode=Inline
  pct2mm2 : Subsystem  TreatAsAtomicUnit=on
      settings: RTWSystemCode=Inline
  VINP_EDUSynchPosn_mm : Outport  OutDataType=sfix(16)  OutScaling=2^0
  VINP_EDUSynchPosnValid_flg : Outport  Port=2  OutDataType=sfix(16)  OutScaling=2^0
  wires:
  Gain/1 -> pct2mm1/1(gain3)
  Constant2/1 -> Gain/1
  VINP_EDUSynchPosnPWMDC_pct/1 -> pct2mm1/2(VINP_EDUSynchPosnPWMDC_pct)
  Switch1/1 -> VINP_EDUSynchPosnValid_flg/1  "VINP_EDUSynchPosnValid_flg"
  Logical Operator1/1 -> Logical Operator/2
  Logical Operator/1 -> Switch2/2
  Switch2/1 -> VINP_EDUSynchPosn_mm/1  "VINP_EDUSynchPosn_mm"
  pct2mm2/1(VINP_EDUSynchPosnPWMKDC_mm) -> Switch2/1  "VINP_EDUSynchPosnPWMKDC_mm"
  pct2mm1/1(VINP_EDUSynchPosnPWMDC_mm) -> Switch2/3  "VINP_EDUSynchPosnPWMDC_mm"
  VINP_EDUSynchPosnPWMKDC_pct/1 -> pct2mm2/2(VINP_EDUSynchPosnPWMKDC_pct)
  VINP_EDUSynchPosnPWMKDCValid_flg/1 -> Switch1/1, Logical Operator2/1, Logical Operator/1
  VINP_EDUSynchPosnPWMDCValid_flg/1 -> Switch1/3, Logical Operator3/1, Logical Operator1/1
  Logical Operator3/1 -> Logical Operator2/2
  Logical Operator2/1 -> Switch1/2
  cnst_EDUSynchDisp/1 -> pct2mm2/1(gain1)

== system inp/INP/Pre-Process/BINP_ouputs_5ms/Signal Process/VehSpdRaw_Calc ==
  VINP_EDUOutputShaftSpdRaw_rpm : Inport
  VINP_VehSpdRawABS_kph : Inport  Port=2
  VINP_TMSpd_rpm : Inport  Port=3
  VINP_EDUOutputShaftSpdRawValid_flg : Inport  Port=4
  Compare To Constant : simulink/Logic and Bit Operations/Compare To Constant  SystemSampleTime=-1  relop=>=  const=0  LogicOutDataTypeMode=uint8
  Hysteresis : hcu_lib/Hysteresis  SystemSampleTime=-1
  Product : Product  OutDataType=fixdt(1, 16)  OutScaling=2^0  RndMeth=Zero
  Relational Operator : RelationalOperator  Operator=>  LogicOutDataTypeMode=boolean  LogicDataType=fixdt(0, 8)  OutDataTypeStr=boolean
  Switch{,1..3} (4 alike) : Switch  Criteria=u2 ~= 0  Threshold=0.5  OutDataType=fixdt(1, 16)  OutScaling=2^0
  Unit Delay : UnitDelay  X0=1  SampleTime=-1
  cnst_EDUSynchDisp : Constant  Value=KINP_VehSpdSigKeepThres_kph  OutDataType=fixdt(1, 16)  OutScaling=2^0
  cnst_EDUSynchDisp1 : Constant  Value=KINP_TMSpd2VehSpdSigNeg_rpm  OutDataType=fixdt(1, 16)  OutScaling=2^0
  cnst_EDUSynchDisp2 : Constant  Value=KINP_TMSpd2VehSpdSigPos_rpm  OutDataType=fixdt(1, 16)  OutScaling=2^0
  cnst_EDUSynchDisp3 : Constant  OutDataTypeMode=single  OutDataType=fixdt(1, 16)  OutScaling=2^0  OutDataTypeStr=single
  cnst_EDUSynchDisp4 : Constant  Value=-1  OutDataTypeMode=single  OutDataType=fixdt(1, 16)  OutScaling=2^0  OutDataTypeStr=single
  cnst_EDUSynchDisp5 : Constant  OutDataTypeMode=single  OutDataType=fixdt(1, 16)  OutScaling=2^0  OutDataTypeStr=single
  cnst_EDUSynchDisp6 : Constant  Value=-1  OutDataTypeMode=single  OutDataType=fixdt(1, 16)  OutScaling=2^0  OutDataTypeStr=single
  VINP_VehSpdRaw_kph : Outport
  wires:
  VINP_TMSpd_rpm/1 -> Hysteresis/1
  Product/1 -> VINP_VehSpdRaw_kph/1  "VINP_VehSpdRaw_kph"
  VINP_EDUOutputShaftSpdRawValid_flg/1 -> Switch2/2
  VINP_EDUOutputShaftSpdRaw_rpm/1 -> Compare To Constant/1
  [VINP_VehSpdRawABS_kph] -> Product/2
  Switch2/1 -> Product/1
  Switch3/1 -> Switch2/1
  cnst_EDUSynchDisp6/1 -> Switch3/3
  Compare To Constant/1 -> Switch3/2
  cnst_EDUSynchDisp5/1 -> Switch3/1
  Switch1/1 -> Switch/3
  cnst_EDUSynchDisp4/1 -> Switch1/3
  Hysteresis/1 -> Switch1/2
  cnst_EDUSynchDisp3/1 -> Switch1/1
  Unit Delay/1 -> Switch/1
  Switch/1 -> Switch2/3, Unit Delay/1
  Relational Operator/1 -> Switch/2
  cnst_EDUSynchDisp1/1 -> Hysteresis/3
  cnst_EDUSynchDisp2/1 -> Hysteresis/2
  cnst_EDUSynchDisp/1 -> Relational Operator/2
  VINP_VehSpdRawABS_kph/1 -> [VINP_VehSpdRawABS_kph], Relational Operator/1

== system inp/INP/Pre-Process/BINP_ouputs_5ms/Signal Process/VehSpd_Calc ==
  VINP_EDUOutputShaftSpdRaw_rpm : Inport  OutDataType=sfix(16)  OutScaling=2^0
  <VINP_VehSpdRaw_kph> : Inport  Port=2  OutDataType=sfix(16)  OutScaling=2^0
  VINP_EDUOutputShaftSpdRawValid_flg : Inport  Port=3  OutDataType=sfix(16)  OutScaling=2^0
  <VINP_VehSpdRawValid_flg> : Inport  Port=4  OutDataType=sfix(16)  OutScaling=2^0
  KPH2RPM : Subsystem
  Logical Operator{,2,4,6} (4 alike) : Logic  AllPortsSameDT=off  OutDataTypeMode=boolean  OutDataTypeStr=boolean
  Logical Operator{1,3,5,7} (4 alike) : Logic  Operator=NOT  AllPortsSameDT=off  OutDataTypeMode=boolean  OutDataTypeStr=boolean
  RPM2KPH : Subsystem
  Switch{1..4} (4 alike) : Switch  Criteria=u2 ~= 0  Threshold=0.5  OutDataType=sfix(16)  OutScaling=2^0
  VINP_VehSpd_kph : Outport  OutDataType=sfix(16)  OutScaling=2^0
  VINP_EDUOutputShaftSpd_rpm : Outport  Port=2  OutDataType=sfix(16)  OutScaling=2^0
  VINP_VehSpdValid_flg : Outport  Port=3  OutDataType=sfix(16)  OutScaling=2^0
  VINP_EDUOutputShaftSpdValid_flg : Outport  Port=4  OutDataType=sfix(16)  OutScaling=2^0
  wires:
  <VINP_VehSpdRaw_kph>/1 -> Switch2/3, KPH2RPM/1(KPH)
  Switch2/1 -> VINP_VehSpd_kph/1  "VINP_VehSpd_kph"
  Logical Operator1/1 -> Logical Operator/2
  VINP_EDUOutputShaftSpdRawValid_flg/1 -> [VINP_EDUOutputShaftSpdRawValid_flg], Logical Operator/1
  <VINP_VehSpdRawValid_flg>/1 -> [VINP_VehSpdRawValid_flg], Logical Operator2/1, Logical Operator1/1
  VINP_EDUOutputShaftSpdRaw_rpm/1 -> [VINP_EDUOutputShaftSpdRaw_rpm], RPM2KPH/1(RPM)
  Logical Operator/1 -> Switch2/2
  Switch1/1 -> VINP_EDUOutputShaftSpd_rpm/1  "VINP_EDUOutputShaftSpd_rpm"
  Logical Operator2/1 -> Switch1/2
  Logical Operator3/1 -> Logical Operator2/2
  [VINP_EDUOutputShaftSpdRawValid_flg] -> Logical Operator3/1
  [VINP_EDUOutputShaftSpdRaw_rpm] -> Switch1/3
  Switch3/1 -> VINP_VehSpdValid_flg/1  "VINP_VehSpdValid_flg"
  Logical Operator5/1 -> Logical Operator4/2
  [VINP_EDUOutputShaftSpdRawValid_flg] -> Switch4/3, Logical Operator7/1, Switch3/1, Logical Operator4/1
  [VINP_VehSpdRawValid_flg] -> Switch3/3, Logical Operator6/1, Switch4/1, Logical Operator5/1
  Logical Operator4/1 -> Switch3/2
  Switch4/1 -> VINP_EDUOutputShaftSpdValid_flg/1  "VINP_EDUOutputShaftSpdValid_flg"
  Logical Operator6/1 -> Switch4/2
  Logical Operator7/1 -> Logical Operator6/2
  RPM2KPH/1(KPH) -> Switch2/1
  KPH2RPM/1(RPM) -> Switch1/1

== system inp/INP/Pre-Process/BINP_ouputs_5ms/Signal Process/SynchPosn/pct2mm1 ==
  gain3 : Inport  OutDataType=sfix(16)  OutScaling=2^0
  VINP_EDUSynchPosnPWMDC_pct : Inport  Port=2  OutDataType=sfix(16)  OutScaling=2^0
  Product_tmp3 : Product  Tag=struct('comment',struct('text','','placement',1),'logdata',struct('maxnumvals',inf,'plotchannels',[],'stepsize',0,'downsampling',1,'loggingmode',3,'channels',1),'output',struct('width',1,'name','$S_$B','unit','','type','Int32Bin15','offset',0,'max',65535,'min',-65536,'freeze',1,'lsb',2^-15,'arb',0,'class','default','address','','description','','autoscalingmode',1,'lowerheadroom',1,'upperheadroom',1,'headroomunit','bit','checkmin',0,'checkmax',0,'show',0),'inputs','**','exceptionhandling',1,'date',731455.58640515)  Inputs=**/  OutDataType=sfix(16)  OutScaling=2^0  RndMeth=Zero  InputSameDT=on  OutDataTypeStr=Inherit: Same as first input
  Sum2 : Sum  Tag=struct('comment',struct('text','','placement',1),'logdata',struct('maxnumvals',inf,'plotchannels',[],'stepsize',0,'downsampling',1,'loggingmode',3,'channels',1),'output',struct('width',1,'name','$S_$B','unit','','type','Int32Bin15','offset',0,'max',65535,'min',-65536,'freeze',1,'lsb',2^-15,'arb',0,'class','default','address','','description','','autoscalingmode',1,'lowerheadroom',1,'upperheadroom',1,'headroomunit','bit','checkmin',0,'checkmax',0,'show',0),'inputs','-+','date',731455.586330463)  Inputs=+-  OutDataType=sfix(16)  OutScaling=2^0  InputSameDT=on  OutDataTypeStr=Inherit: Same as first input
  zero1 : Constant  Tag=struct('comment',struct('text','','placement',1),'output',struct('width',1,'name','$S_$B','unit','','type','Int16','offset',0,'max',NaN,'min',NaN,'freeze',1,'lsb',1,'arb',0,'class','default','address','','description','','value','0','tolerance',1,'show',0),'date',731455.58675544)  Value=80  OutDataTypeMode=single  OutDataType=sfix(16)  OutScaling=2^0  OutDataTypeStr=single
  zero9 : Constant  Tag=struct('comment',struct('text','','placement',1),'output',struct('width',1,'name','$S_$B','unit','','type','Int16','offset',0,'max',NaN,'min',NaN,'freeze',1,'lsb',1,'arb',0,'class','default','address','','description','','value','0','tolerance',1,'show',0),'date',731455.58675544)  Value=50  OutDataTypeMode=single  OutDataType=sfix(16)  OutScaling=2^0  OutDataTypeStr=single
  VINP_EDUSynchPosnPWMDC_mm : Outport  OutDataType=sfix(16)  OutScaling=2^0
  wires:
  zero1/1 -> Product_tmp3/3
  Product_tmp3/1 -> VINP_EDUSynchPosnPWMDC_mm/1
  gain3/1 -> Product_tmp3/2
  Sum2/1 -> Product_tmp3/1
  zero9/1 -> Sum2/2
  VINP_EDUSynchPosnPWMDC_pct/1 -> Sum2/1

== system inp/INP/Pre-Process/BINP_ouputs_5ms/Signal Process/SynchPosn/pct2mm2 ==
  gain1 : Inport  OutDataType=sfix(16)  OutScaling=2^0
  VINP_EDUSynchPosnPWMKDC_pct : Inport  Port=2  OutDataType=sfix(16)  OutScaling=2^0
  Product_tmp1 : Product  Tag=struct('comment',struct('text','','placement',1),'logdata',struct('maxnumvals',inf,'plotchannels',[],'stepsize',0,'downsampling',1,'loggingmode',3,'channels',1),'output',struct('width',1,'name','$S_$B','unit','','type','Int32Bin15','offset',0,'max',65535,'min',-65536,'freeze',1,'lsb',2^-15,'arb',0,'class','default','address','','description','','autoscalingmode',1,'lowerheadroom',1,'upperheadroom',1,'headroomunit','bit','checkmin',0,'checkmax',0,'show',0),'inputs','**','exceptionhandling',1,'date',731455.58640515)  Inputs=**/  OutDataType=sfix(16)  OutScaling=2^0  RndMeth=Zero  InputSameDT=on  OutDataTypeStr=Inherit: Same as first input
  Sum : Sum  Tag=struct('comment',struct('text','','placement',1),'logdata',struct('maxnumvals',inf,'plotchannels',[],'stepsize',0,'downsampling',1,'loggingmode',3,'channels',1),'output',struct('width',1,'name','$S_$B','unit','','type','Int32Bin15','offset',0,'max',65535,'min',-65536,'freeze',1,'lsb',2^-15,'arb',0,'class','default','address','','description','','autoscalingmode',1,'lowerheadroom',1,'upperheadroom',1,'headroomunit','bit','checkmin',0,'checkmax',0,'show',0),'inputs','-+','date',731455.586330463)  Inputs=+-  OutDataType=sfix(16)  OutScaling=2^0  InputSameDT=on  OutDataTypeStr=Inherit: Same as first input
  zero1 : Constant  Tag=struct('comment',struct('text','','placement',1),'output',struct('width',1,'name','$S_$B','unit','','type','Int16','offset',0,'max',NaN,'min',NaN,'freeze',1,'lsb',1,'arb',0,'class','default','address','','description','','value','0','tolerance',1,'show',0),'date',731455.58675544)  Value=80  OutDataTypeMode=single  OutDataType=sfix(16)  OutScaling=2^0  OutDataTypeStr=single
  zero9 : Constant  Tag=struct('comment',struct('text','','placement',1),'output',struct('width',1,'name','$S_$B','unit','','type','Int16','offset',0,'max',NaN,'min',NaN,'freeze',1,'lsb',1,'arb',0,'class','default','address','','description','','value','0','tolerance',1,'show',0),'date',731455.58675544)  Value=50  OutDataTypeMode=single  OutDataType=sfix(16)  OutScaling=2^0  OutDataTypeStr=single
  VINP_EDUSynchPosnPWMKDC_mm : Outport  OutDataType=sfix(16)  OutScaling=2^0
  wires:
  zero1/1 -> Product_tmp1/3
  Product_tmp1/1 -> VINP_EDUSynchPosnPWMKDC_mm/1
  gain1/1 -> Product_tmp1/2
  Sum/1 -> Product_tmp1/1
  zero9/1 -> Sum/2
  VINP_EDUSynchPosnPWMKDC_pct/1 -> Sum/1

== system inp/INP/Pre-Process/BINP_ouputs_5ms/Signal Process/VehSpd_Calc/KPH2RPM ==
  KPH : Inport
  Constant1 : Constant  Value=MIN2SEC  OutDataType=fixdt(1, 16)  OutScaling=2^0
  Constant2 : Constant  Value=2  OutDataTypeMode=single  OutDataType=fixdt(1, 16)  OutScaling=2^0  OutDataTypeStr=single
  Constant3 : Constant  Value=PI  OutDataType=fixdt(1, 16)  OutScaling=2^0
  Constant4 : Constant  Value=TIRE_RADIUS  OutDataType=fixdt(1, 16)  OutScaling=2^0
  Constant5 : Constant  Value=KPH2MPS  OutDataType=fixdt(1, 16)  OutScaling=2^0
  Product : Product  Inputs=**///*  OutDataType=fixdt(1, 16)  OutScaling=2^0  RndMeth=Zero
  RPM : Outport
  wires:
  Product/1 -> RPM/1
  KPH/1 -> Product/1
  Constant5/1 -> Product/2
  Constant2/1 -> Product/3
  Constant3/1 -> Product/4
  Constant4/1 -> Product/5
  Constant1/1 -> Product/6

== system inp/INP/Pre-Process/BINP_ouputs_5ms/Signal Process/VehSpd_Calc/RPM2KPH ==
  RPM : Inport
  Constant1 : Constant  Value=MIN2SEC  OutDataType=fixdt(1, 16)  OutScaling=2^0
  Constant2 : Constant  Value=2  OutDataTypeMode=single  OutDataType=fixdt(1, 16)  OutScaling=2^0  OutDataTypeStr=single
  Constant3 : Constant  Value=PI  OutDataType=fixdt(1, 16)  OutScaling=2^0
  Constant4 : Constant  Value=TIRE_RADIUS  OutDataType=fixdt(1, 16)  OutScaling=2^0
  Constant5 : Constant  Value=MPS2KPH  OutDataType=fixdt(1, 16)  OutScaling=2^0
  Product : Product  Inputs=*/****  OutDataType=fixdt(1, 16)  OutScaling=2^0  RndMeth=Zero
  KPH : Outport
  wires:
  RPM/1 -> Product/1
  Product/1 -> KPH/1
  Constant1/1 -> Product/2
  Constant2/1 -> Product/3
  Constant3/1 -> Product/4
  Constant4/1 -> Product/5
  Constant5/1 -> Product/6

== stateflow chart INP/Chart ==
  (default) -> (junction 3) : {
      | trig_5ms_raw;
      | trig_sig_chk_5ms;
      | trig_sig_chk_10ms;
      | trig_sig_chk_100ms;
      | }
  events: trig_5ms_raw output FUNCTION_CALL_EVENT; trig_sig_chk_5ms output FUNCTION_CALL_EVENT; event_5ms_trig input FUNCTION_CALL_EVENT; trig_sig_chk_10ms output FUNCTION_CALL_EVENT; trig_sig_chk_100ms output FUNCTION_CALL_EVENT

== stateflow chart INP/INP_5MS/HW_HCU_5ms/Subsys VINP_EDUSynchPosnPWMDC_pct/rff_ctl ==
  (default) -> (junction 12)
  (junction 12) -> (junction 16) [order 2] : {count-=dec;}
  (junction 12) -> (junction 16) [order 1] : [i_fault]
      | {count+=inc;}
  (junction 13) -> (junction 14) [order 1] : [count>=sat]
      | {count=sat;
      | fault_flg=1;}
  (junction 13) -> (junction 14) [order 2] : [count<=0]
      | {count=0;
      | fault_flg=0;}
  (junction 13) -> (junction 14) [order 3]
  (junction 14) -> (junction 15) : {ff_count = count;}
  (junction 16) -> (junction 13)
  data: sat input uint8; inc input uint8; dec input uint8; i_fault input boolean; fault_flg output boolean =0; ff_count output uint8; count local int16

== stateflow chart INP/Chart1 ==
  (default) -> (junction 34) : {
      | trig_inp_raw_10ms;
      | trig_can_msg_alive_10ms;
      | }
  events: event_10ms_trig input FUNCTION_CALL_EVENT; trig_inp_raw_10ms output FUNCTION_CALL_EVENT; trig_can_msg_alive_10ms output FUNCTION_CALL_EVENT
